simulink model "passiveBalancing"  (R2020b)
settings: Solver=ode23t  StartTime=0.0  StopTime=3600 * 15  MaxStep=.5  RelTol=1e-3  AbsTol=1e-3  EnableMultiTasking=on
PreLoadFcn:
  | passiveBalancing_ini;
model workspace (MAT data in the model file):
  Switch = 1
values from neighbouring files (symbols this model uses):
  I_cc = 4    [passiveBalancing_ini.m]
  I_gain = 10    [passiveBalancing_ini.m]
  P_gain = 100    [passiveBalancing_ini.m]
  R_bleed = 20    [passiveBalancing_ini.m]
  T_f = 600    [passiveBalancing_ini.m]
  V_top = 4.1    [passiveBalancing_ini.m]
libraries: fl_lib x15, nesl_utility x15, ee_lib x6, simulink x1, pid_lib x1
(part 2 of 2)

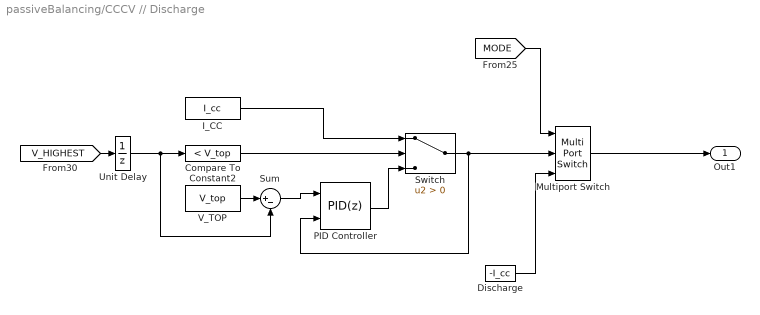
== system passiveBalancing/CCCV // Discharge ==
  Compare To Constant2 : simulink/Logic and Bit Operations/Compare To Constant  relop=<  const=V_top  OutDataTypeStr=boolean
  Discharge : Constant  Value=-I_cc
  I_CC : Constant  Value=I_cc
  Multiport Switch : MultiPortSwitch  DataPortOrder=Specify indices  DataPortIndices={1,2}  DiagnosticForDefault=None
  PID Controller : pid_lib/PID Controller  Controller=PID  Form=Parallel  TimeDomain=Discrete-time  UseExternalTs=off  SampleTime=1  IntegratorMethod=Forward Euler  FilterMethod=Forward Euler  ControllerParametersSource=internal  P=P_gain  I=I_gain  D=0  UseFilter=on  N=100  TunerSelectOption=Transfer Function Based (PID Tuner App)  InitialConditionSource=internal  InitialConditionForIntegrator=10  InitialConditionForFilter=0  DifferentiatorICPrevScaledInput=0  ExternalReset=none  TrackingMode=on  Kt=1  LimitOutput=on  SatLimitsSource=internal  UpperSaturationLimit=Inf  LowerSaturationLimit=0  LinearizeAsGain=on  AntiWindupMode=clamping  Kb=1  POutMin=[]  POutMax=[]  IOutMin=[]  IOutMax=[]  DOutMin=[]  DOutMax=[]  NOutMin=[]  NOutMax=[]  SumOutMin=[]  SumOutMax=[]  SaturationOutMin=[]  SaturationOutMax=[]  PParamMin=[]  PParamMax=[]  IParamMin=[]  IParamMax=[]  DParamMin=[]  DParamMax=[]  NParamMin=[]  NParamMax=[]  KbParamMin=[]  KbParamMax=[]  KtParamMin=[]  KtParamMax=[]  KbOutMin=[]  KbOutMax=[]  KtOutMin=[]  KtOutMax=[]  IntegratorOutMin=[]  IntegratorOutMax=[]  FilterOutMin=[]  FilterOutMax=[]  SumI1OutMin=[]  SumI1OutMax=[]  SumI2OutMin=[]  SumI2OutMax=[]  SumI3OutMin=[]  SumI3OutMax=[]  SumI4OutMin=[]  SumI4OutMax=[]  SumDOutMin=[]  SumDOutMax=[]  DifferentiatorOutMin=[]  DifferentiatorOutMax=[]  FilterDiffOutCoefMin=[]  FilterDiffOutCoefMax=[]  ReciprocalOutMin=[]  ReciprocalOutMax=[]  SumDenOutMin=[]  SumDenOutMax=[]  SumNumOutMin=[]  SumNumOutMax=[]  DivideOutMin=[]  DivideOutMax=[]  UdiffTsProdOutMin=[]  UdiffTsProdOutMax=[]  NTsProdOutMin=[]  NTsProdOutMax=[]  UintegralTsProdOutMin=[]  UintegralTsProdOutMax=[]  UngainTsProdOutMin=[]  UngainTsProdOutMax=[]  IntegratorContinuousStateAttributes=''  IntegratorStateMustResolveToSignalObject=off  IntegratorRTWStateStorageClass=Auto  FilterContinuousStateAttributes=''  FilterStateMustResolveToSignalObject=off  FilterRTWStateStorageClass=Auto  ParallelPVariant=InternalParameters  IdealPVariant=Disabled  IVariant=InternalParameters  DVariant=InternalParameters  IntegratorVariant=Discrete  SatVariant=Enabled  AWVariant=DiscClampingParallel  PCopyVariant=Disabled  TRVariant=Enabled  FdbkBlocksVariant=Forward  IdealPFdbkVariant=Disabled  SatFdbkVariant=Disabled  DerivativeFilterVariant=ForwardEulerFilter  NVariant=InternalParameters  NCopyVariant=Disabled  FilterICVariant=InternalICsFilter  IntegratorICVariant=InternalICs  ExternalResetVariant=Disabled  TRSumVariant=TrackingMode  SumFdbkVariant=Disabled  SumVariant=Sum_PID  TsampFilterVariant=InternalTs  TsampNgainVariant=Passthrough  TsampIntegralVariant=Passthrough  ExternalSaturationOutDataTypeStr=Inherit: Same as second input
  Sum : Sum  Inputs=|+-
  Switch : Switch  Criteria=u2 > Threshold
  Unit Delay : UnitDelay  SampleTime=-1  HasFrameUpgradeWarning=on
  V_TOP : Constant  Value=V_top
  Out1 : Outport
  wires:
  Switch/1 -> PID Controller/2, Multiport Switch/2
  Compare To Constant2/1 -> Switch/2
  Unit Delay/1 -> Sum/2, Compare To Constant2/1
  I_CC/1 -> Switch/1
  PID Controller/1 -> Switch/3
  Sum/1 -> PID Controller/1
  [MODE] -> Multiport Switch/1
  V_TOP/1 -> Sum/1
  [V_HIGHEST] -> Unit Delay/1
  Discharge/1 -> Multiport Switch/3
  Multiport Switch/1 -> Out1/1

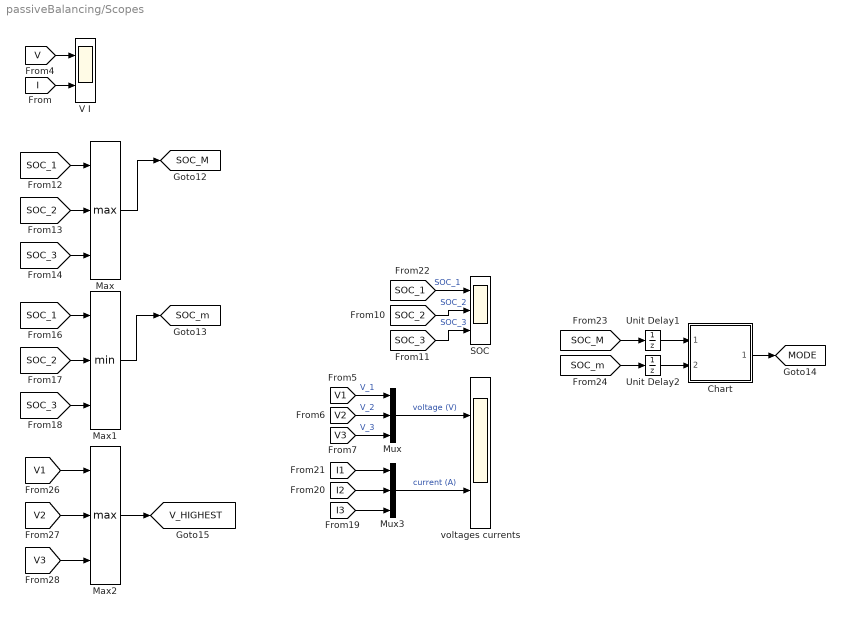
== system passiveBalancing/Scopes ==
  Chart : Stateflow chart  TreatAsAtomicUnit=on
  Max : MinMax  Function=max  Inputs=3
  Max1 : MinMax  Inputs=3
  Max2 : MinMax  Function=max  Inputs=3
  Mux : Mux  Inputs=3
  Mux3 : Mux  Inputs=3
  SOC : Scope  NumInputPorts=3
  Unit Delay1 : UnitDelay  InitialCondition=1  SampleTime=-1  HasFrameUpgradeWarning=on
  Unit Delay2 : UnitDelay  InitialCondition=1  SampleTime=-1  HasFrameUpgradeWarning=on
  V I : Scope  NumInputPorts=2
  voltages currents : Scope  NumInputPorts=2
  tag scope: MODE=global, SOC_M=global, SOC_m=global, V_HIGHEST=global
  wires:
  [V3] -> Mux/3  "V_3"
  [SOC_3] -> SOC/3  "SOC_3"
  [I2] -> Mux3/2
  [SOC_1] -> SOC/1  "SOC_1"
  [I1] -> Mux3/1
  [I3] -> Mux3/3
  Mux/1 -> voltages currents/1  "voltage (V)"
  [V2] -> Mux/2  "V_2"
  Max2/1 -> [V_HIGHEST]
  [V] -> V I/1
  [SOC_3] -> Max/3
  Max1/1 -> [SOC_m]
  [V2] -> Max2/2
  [SOC_2] -> Max/2
  [V1] -> Max2/1
  Max/1 -> [SOC_M]
  [SOC_2] -> Max1/2
  [SOC_2] -> SOC/2  "SOC_2"
  [V1] -> Mux/1  "V_1"
  [SOC_1] -> Max1/1
  Mux3/1 -> voltages currents/2  "current (A)"
  [V3] -> Max2/3
  [SOC_1] -> Max/1
  [I] -> V I/2
  [SOC_3] -> Max1/3
  [SOC_m] -> Unit Delay2/1
  Unit Delay1/1 -> Chart/1(SOC_MAX)
  [SOC_M] -> Unit Delay1/1
  Unit Delay2/1 -> Chart/2(SOC_min)
  Chart/1(MODE) -> [MODE]

== stateflow chart passiveBalancing/balancing logic ==
  state finish
    entry: s1 = 0;
    s2 = 0;
    s3 = 0;
  state init
    entry: s1 = 0;
    s2 = 0;
    s3 = 0;
  state balancing
    during: lowest = lowestCell(v1,v2,v3);
    state cell3_low
      entry: s1 = 1;
      s2 = 1;
      s3 = 0;
      exit: s1 = 0;
      s2 = 0;
      s3 = 0;
    state cell2_low
      entry: s1 = 1;
      s3 = 1;
      s2 = 0;
      exit: s1 = 0;
      s3 = 0;
      s2 = 0;
    state cell1_low
      entry: s2 = 1;
      s3 = 1;
      s1 = 0;
      exit: s1 = 0;
      s3 = 0;
      s2 = 0;
    (default) -> (junction 382) : {lowest = lowestCell(v1,v2,v3);}
    (junction 382) -> cell3_low [order 1] : [lowest==3]
    (junction 382) -> cell1_low [order 2] : [lowest==1]
    (junction 382) -> cell2_low [order 3] : [lowest==2]
    cell2_low -> cell1_low [order 2] : [lowest==1]
    cell3_low -> cell2_low [order 1] : [lowest==2]
    cell2_low -> cell3_low [order 1] : [lowest==3]
    cell1_low -> cell2_low [order 1] : [lowest==2]
    cell3_low -> cell1_low [order 2] : [lowest==1]
    cell1_low -> cell3_low [order 2] : [lowest==3]
  (default) -> init
  finish -> balancing : [abs(max([v1 v2 v3]) - min([v1 v2 v3])) > dV && after(1,sec)]
  balancing -> finish : [abs(max([v1 v2 v3]) - min([v1 v2 v3])) < dV]
  init -> balancing : [abs(max([v1 v2 v3]) - min([v1 v2 v3])) > dV]
  data: a function_input; b function_input; c function_input; lowidx function_output; v1 input; v2 input; v3 input; s1 output; s2 output; s3 output; dV parameter; lowest local
  function lowidx = lowestCell(a,b,c):
    | function lowidx = lowestCell(a,b,c)
    | [~,k] = sort([a,b,c],'ascend');
    | lowidx = k(1);

== stateflow chart passiveBalancing/Scopes/Chart ==
  state wait
  state DISCHARGE
    during: MODE = 2;
  state CHARGE
    during: MODE = 1;
  (default) -> wait
  wait -> (junction 14)
  (junction 14) -> (junction 16) [order 1] : [SOC_MAX<0.5]
  (junction 14) -> DISCHARGE [order 2] : [SOC_MAX>=0.5]
  (junction 16) -> (junction 19)
  CHARGE -> DISCHARGE : [SOC_MAX > 0.99 || after(5000,sec)]
  DISCHARGE -> CHARGE : [SOC_min < 0.3]
  (junction 19) -> CHARGE
  data: MODE output; SOC_MAX input; SOC_min input
